simulink model "ex3"  (R2016a)
settings: Solver=VariableStepDiscrete  SolverMode=SingleTasking  StartTime=0.0  StopTime=1  RelTol=1e-3
model workspace (MAT data in the model file):
  M = 4
libraries: dspindex x4, commcnvcod2 x2, commdigbbndpm3 x2, dspxfrm3 x2, commchan3 x1, commrandsrc3 x1, commsink2 x1
settings Model: Creator=gvkk1  LastModifiedBy=gvkk1
settings DataIOCC: LimitDataPoints=on  SaveOutput=off  SaveTime=off
settings OptimizationCC: BooleanDataType=off  DefaultParameterBehavior=Inlined  LocalBlockOutputs=off
settings DebuggingCC: AlgebraicLoopMsg=error  SingleTaskRateTransMsg=error  AllowSymbolicDim=off
settings ConfigComp: CovModelRefEnable=Off  CovSFcnEnable=off

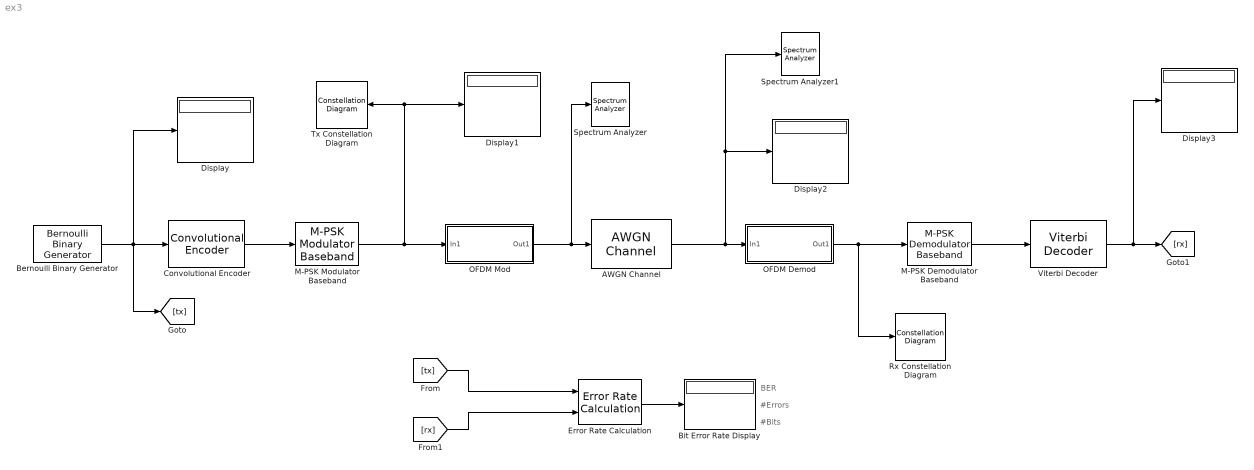
== system ex3 ==
  note: BER
  note: #Bits
  note: #Errors
  AWGN Channel : commchan3/AWGN Channel  InputProcessing=Columns as channels (frame based)  seed=67  noiseMode="Signal to noise ratio  (SNR)"  EbNodB=10  EsNodB=10  SNRdB=30  bitsPerSym=2  Ps=1  Tsym=1  variance=1
  Bernoulli Binary Generator : commrandsrc3/Bernoulli Binary Generator  ProbabilityOfZero=0.5  SeedSource=Auto  Seed=0  SampleTime=(8e-6)/64  SamplesPerFrame=48  OutputDataType=boolean  SimulateUsing=Interpreted execution
  Bit Error Rate Display : Display
  Convolutional Encoder : commcnvcod2/Convolutional Encoder  trellis=poly2trellis(7, [171 133])  opMode=Truncated (reset every frame)  DelayedResetAction=off  hasIniStPort=off  hasFinStPort=off  usePuncVector=off  punctureVector=[1; 1; 0; 1; 0; 1]  reset=Unused parameter value
  Display{,1..3} (4 alike) : Display
  Error Rate Calculation : commsink2/Error Rate Calculation  N=0  st_delay=0  cp_mode=Entire frame  subframe=[]  PMode=Port  WsName=ErrorVec  RsMode2=off  stop=off  numErr=100  maxBits=1e6
  M-PSK Demodulator Baseband : commdigbbndpm3/M-PSK Demodulator Baseband  M=M  OutType=Bit  DecType=Hard decision  VarSource=Dialog  Variance=1  Dec=User-defined  Mapping=[3 1 0 2]  Ph=pi/M  outDtype1=Inherit via internal rule  outDtype2=Inherit via internal rule  derotateFactorWordLen=16  derotateFactorDataTypeStr=Inherit: Same word length as input  derotateFactorLastDataTypeStr=Inherit: Same word length as input
  M-PSK Modulator Baseband : commdigbbndpm3/M-PSK Modulator Baseband  M=M  InType=Bit  Enc=User-defined  Mapping=[3 1 0 2]  Ph=pi/M  outDtype=double  outWordLen=16  outUDDataType=sfix(16)  outFracLenMode=Best precision  outFracLen=15  outDataTypeStr=double  outLastDataTypeStr=double
  OFDM Demod : Subsystem
  OFDM Mod : Subsystem
  Rx Constellation Diagram : ConstellationDiagram
  Spectrum Analyzer : SpectrumAnalyzer
  Spectrum Analyzer1 : SpectrumAnalyzer
  Tx Constellation Diagram : ConstellationDiagram
  Viterbi Decoder : commcnvcod2/Viterbi Decoder  trellis=poly2trellis(7, [171 133])  isPunctured=off  punctureVector=[1; 1; 0; 1; 0; 1]  erasures=off  dectype=Hard decision  nsdecb=4  runSigValErrCheck=off  tbdepth=34  opmode=Truncated  reset=off  delayedResetAction=off  smWordLength=16  outDataType=boolean
  wires:
  M-PSK Modulator Baseband/1 -> Display1/1, Tx Constellation Diagram/1, OFDM Mod/1(In1)
  AWGN Channel/1 -> Spectrum Analyzer1/1, Display2/1, OFDM Demod/1(In1)
  [tx] -> Error Rate Calculation/1
  [rx] -> Error Rate Calculation/2
  OFDM Mod/1(Out1) -> AWGN Channel/1, Spectrum Analyzer/1
  OFDM Demod/1(Out1) -> Rx Constellation Diagram/1, M-PSK Demodulator Baseband/1
  Bernoulli Binary Generator/1 -> Convolutional Encoder/1, [tx], Display/1
  M-PSK Demodulator Baseband/1 -> Viterbi Decoder/1
  Viterbi Decoder/1 -> Display3/1, [rx]
  Convolutional Encoder/1 -> M-PSK Modulator Baseband/1
  Error Rate Calculation/1 -> Bit Error Rate Display/1

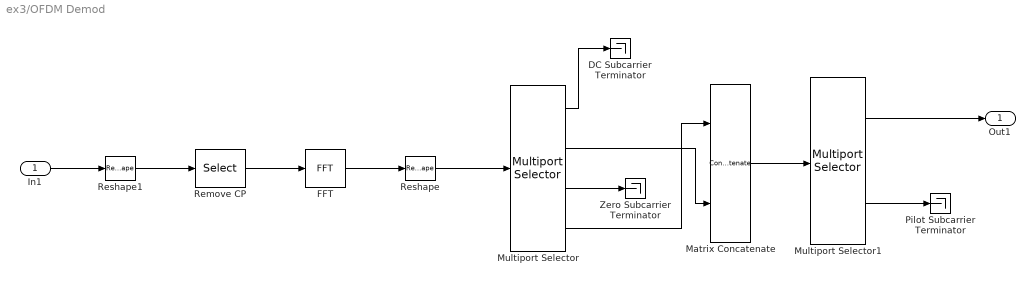
== system ex3/OFDM Demod ==
  In1 : Inport
  DC Subcarrier Terminator : Terminator
  FFT : dspxfrm3/FFT  FFTImplementation=Auto  CompMethod=Table lookup  TableOpt=NEW  TableOptActive=Speed  BitRevOrder=off  Normalize=off  InheritFFTLength=on  FFTLength=64  WrapInput=on  roundingMode=Floor  overflowMode=off  firstCoeffDataTypeStr=Inherit: Same word length as input  firstCoeffLastDataTypeStr=Inherit: Same word length as input  outputMin=[]  outputMax=[]
  Matrix Concatenate : Concatenate  Mode=Multidimensional array
  Multiport Selector : dspindex/Multiport Selector  rowsOrCols=Rows  idxCellArray={1,2:27,28:38,39:64}  idxErrMode=Clip Index
  Multiport Selector1 : dspindex/Multiport Selector  rowsOrCols=Rows  idxCellArray={[1:5 7:19 21:32 34:46 48:52], [6 20 33 47]}  idxErrMode=Clip Index
  Pilot Subcarrier Terminator : Terminator
  Remove CP : Selector  NumberOfDimensions=2  InputPortWidth=3  IndexOptions=Index vector (dialog),Select all  Indices=[17:80],1  OutputSizes=1,1
  Reshape : Reshape  OutputDimensionality=Customize  OutputDimensions=[64, 1]
  Reshape1 : Reshape  OutputDimensionality=Customize  OutputDimensions=[80,1]
  Zero Subcarrier Terminator : Terminator
  Out1 : Outport
  wires:
  In1/1 -> Reshape1/1
  FFT/1 -> Reshape/1
  Remove CP/1 -> FFT/1
  Reshape1/1 -> Remove CP/1
  Reshape/1 -> Multiport Selector/1
  Multiport Selector/1 -> DC Subcarrier Terminator/1
  Multiport Selector/3 -> Zero Subcarrier Terminator/1
  Multiport Selector/2 -> Matrix Concatenate/2
  Multiport Selector/4 -> Matrix Concatenate/1
  Matrix Concatenate/1 -> Multiport Selector1/1
  Multiport Selector1/2 -> Pilot Subcarrier Terminator/1
  Multiport Selector1/1 -> Out1/1

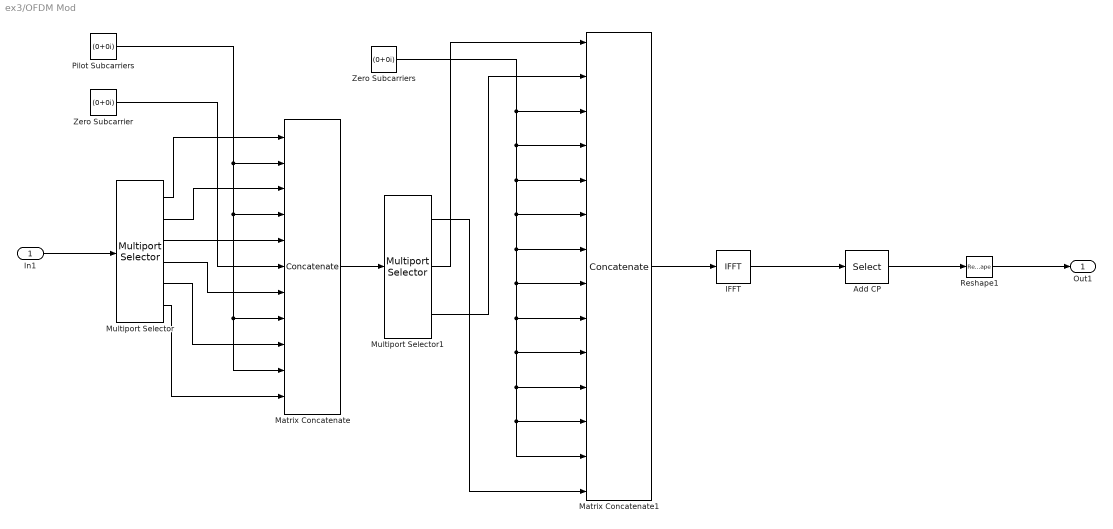
== system ex3/OFDM Mod ==
  In1 : Inport
  Add CP : Selector  NumberOfDimensions=2  InputPortWidth=3  IndexOptions=Index vector (dialog),Select all  Indices=[49:64,1:64],1  OutputSizes=1,1
  IFFT : dspxfrm3/IFFT  FFTImplementation=Auto  CompMethod=Table lookup  TableOpt=NEW  TableOptActive=Speed  BitRevOrder=off  cs_in=off  Normalize=on  InheritFFTLength=on  FFTLength=64  WrapInput=on  mode=Complex  outSamplingMode=Sample based  roundingMode=Floor  overflowMode=off  firstCoeffDataTypeStr=Inherit: Same word length as input  firstCoeffLastDataTypeStr=Inherit: Same word length as input  outputMin=[]  outputMax=[]
  Matrix Concatenate : Concatenate  NumInputs=11  Mode=Multidimensional array
  Matrix Concatenate1 : Concatenate  NumInputs=14  Mode=Multidimensional array
  Multiport Selector : dspindex/Multiport Selector  rowsOrCols=Rows  idxCellArray={1:5, 6:18, 19:24, 25:30, 31:43, 44:48}  idxErrMode=Clip Index
  Multiport Selector1 : dspindex/Multiport Selector  rowsOrCols=Rows  idxCellArray={1:26,27, 28:53}  idxErrMode=Clip Index
  Pilot Subcarriers : Constant  Value=(0+0i)
  Reshape1 : Reshape  OutputDimensionality=Column vector (2-D)
  Zero Subcarrier : Constant  Value=(0+0i)
  "Zero Subcarriers " : Constant  Value=(0+0i)
  Out1 : Outport
  wires:
  Matrix Concatenate1/1 -> IFFT/1
  IFFT/1 -> Add CP/1
  Add CP/1 -> Reshape1/1
  Reshape1/1 -> Out1/1
  Multiport Selector/1 -> Matrix Concatenate/1
  Multiport Selector/2 -> Matrix Concatenate/3
  Multiport Selector/3 -> Matrix Concatenate/5
  Multiport Selector/4 -> Matrix Concatenate/7
  Multiport Selector/5 -> Matrix Concatenate/9
  Multiport Selector/6 -> Matrix Concatenate/11
  Pilot Subcarriers/1 -> Matrix Concatenate/2, Matrix Concatenate/4, Matrix Concatenate/10, Matrix Concatenate/8
  Matrix Concatenate/1 -> Multiport Selector1/1
  Multiport Selector1/3 -> Matrix Concatenate1/2
  Multiport Selector1/1 -> Matrix Concatenate1/14
  Multiport Selector1/2 -> Matrix Concatenate1/1
  "Zero Subcarriers "/1 -> Matrix Concatenate1/4, Matrix Concatenate1/5, Matrix Concatenate1/6, Matrix Concatenate1/7, Matrix Concatenate1/8, Matrix Concatenate1/9, Matrix Concatenate1/10, Matrix Concatenate1/11, Matrix Concatenate1/12, Matrix Concatenate1/13, Matrix Concatenate1/3
  In1/1 -> Multiport Selector/1
  Zero Subcarrier/1 -> Matrix Concatenate/6
